simulink model "untitled"  (R2021a)
settings: Solver=VariableStepAuto  StartTime=0.0  StopTime=10.0  RelTol=1e-3
values from neighbouring files (symbols this model uses):
  B = inv(N)    [Para.m]    (also in Parameters.m = inv(N)*[zeros(3);eye(3)])
  dtheta_LMO = sqrt(muy/r_LMO^3)    [Para.m]    (also in Parameters.m)
  hW = [0 h2 0]'    [Para.m]
  I = [10 0 0;0 5 0;0 0 7.5]    [Para.m]    (also in Parameters.m = diag([5 3 6]))
  i0_LMO = pi/6    (= 0.523598775598)    [Para.m]    (also in Parameters.m)
  K = 5    [Para.m]    (also in Parameters.m)
  N = [eye(3) zeros(3);zeros(3) J]    [Dynamics.m]    (also in Para.m; Parameters.m)
  Omega0_LMO = pi/9    (= 0.349065850399)    [Para.m]    (also in Parameters.m)
  P = 10*eye(3)    [Para.m]    (also in Parameters.m)
  R = eye(6)    [Para.m]    (also in Parameters.m = eye(3))
  S = [0 0 0 0.5 0 0;           0 0 0 0 0.5 0;           0 0 0 0 0 0.5;           f41 0 0 0 0 f46;           0 f52 0 0 0 0;           0 0 f63 f64 0 0]    [Para.m]    (also in Parameters.m; crossMatrix.m = [0 -q3 q2;           q3 0 -q1;           -q2 q1 0])
  theta0_LMO = pi/3    (= 1.0471975512)    [Para.m]    (also in Parameters.m)
undefined symbols (not defined in the file or in its folder): F
settings Model: Creator=VTX  LastModifiedBy=VTX

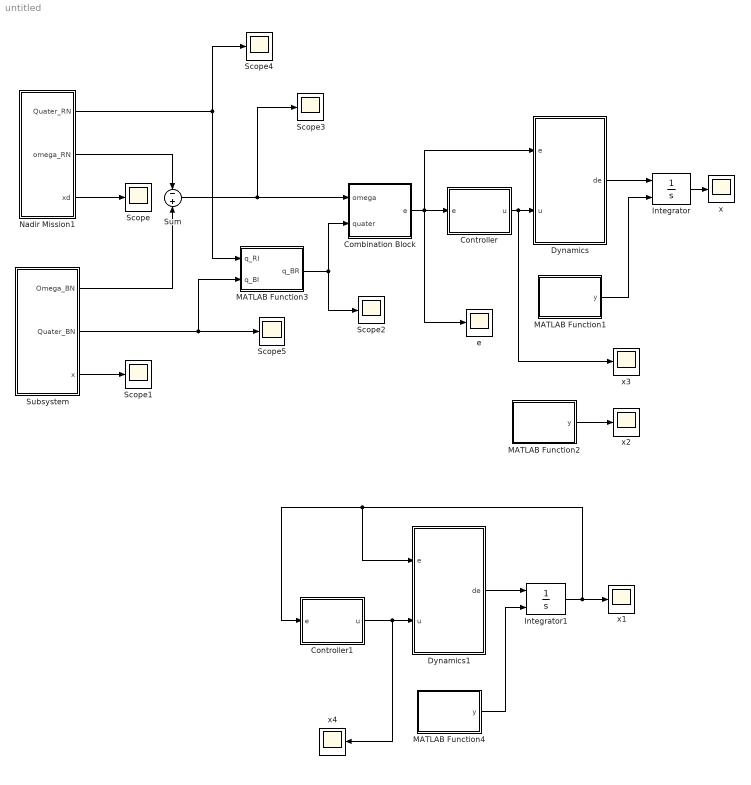
== system untitled ==
  Combination Block : Subsystem
  Controller : MATLAB Function  TreatAsAtomicUnit=on
  Controller1 : MATLAB Function  TreatAsAtomicUnit=on
  Dynamics : MATLAB Function  TreatAsAtomicUnit=on
  Dynamics1 : MATLAB Function  TreatAsAtomicUnit=on
  Integrator : Integrator  InitialConditionSource=external
  Integrator1 : Integrator  InitialConditionSource=external
  MATLAB Function1 : MATLAB Function  TreatAsAtomicUnit=on
  MATLAB Function2 : MATLAB Function  TreatAsAtomicUnit=on
  MATLAB Function3 : MATLAB Function  TreatAsAtomicUnit=on
  MATLAB Function4 : MATLAB Function  TreatAsAtomicUnit=on
  Nadir Mission1 : Subsystem
  Scope{,1..5} (6 alike) : Scope
  Subsystem : Subsystem
  Sum : Sum  Inputs=-|+
  e : Scope
  x{,1..4} (5 alike) : Scope
  wires:
  MATLAB Function2/1(y) -> x2/1
  Integrator1/1 -> Dynamics1/1(e), Controller1/1(e), x1/1
  Dynamics1/1(de) -> Integrator1/1
  MATLAB Function4/1(y) -> Integrator1/2
  Combination Block/1(e) -> e/1, Dynamics/1(e), Controller/1(e)
  Subsystem/1(Omega_BN) -> Sum/2
  Sum/1 -> Combination Block/1(omega), Scope3/1
  Controller1/1(u) -> x4/1, Dynamics1/2(u)
  Dynamics/1(de) -> Integrator/1
  Subsystem/3(x) -> Scope1/1
  MATLAB Function1/1(y) -> Integrator/2
  Nadir Mission1/3(xd) -> Scope/1
  Nadir Mission1/2(omega_RN) -> Sum/1
  Controller/1(u) -> x3/1, Dynamics/2(u)
  Integrator/1 -> x/1
  MATLAB Function3/1(q_BR) -> Combination Block/2(quater), Scope2/1
  Subsystem/2(Quater_BN) -> MATLAB Function3/2(q_BI), Scope5/1
  Nadir Mission1/1(Quater_RN) -> Scope4/1, MATLAB Function3/1(q_RI)

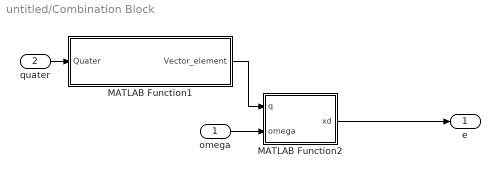
== system untitled/Combination Block ==
  omega : Inport
  quater : Inport  Port=2
  MATLAB Function1 : MATLAB Function  TreatAsAtomicUnit=on
  MATLAB Function2 : MATLAB Function  TreatAsAtomicUnit=on
  e : Outport
  wires:
  MATLAB Function2/1(xd) -> e/1
  MATLAB Function1/1(Vector_element) -> MATLAB Function2/1(q)
  quater/1 -> MATLAB Function1/1(Quater)
  omega/1 -> MATLAB Function2/2(omega)

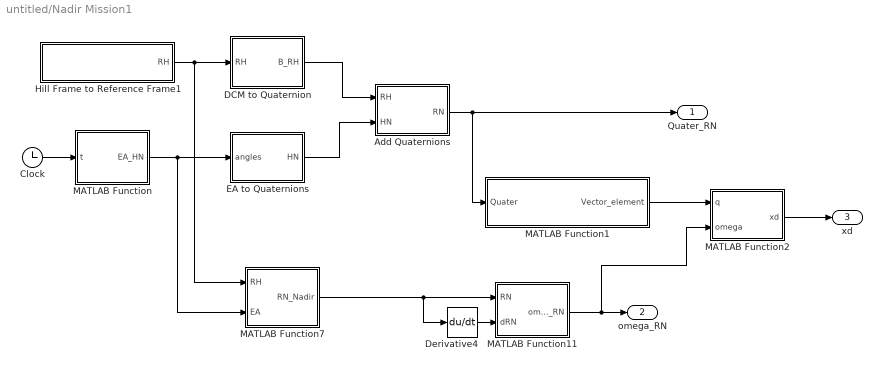
== system untitled/Nadir Mission1 ==
  Add Quaternions : MATLAB Function  TreatAsAtomicUnit=on
  Clock : Clock
  DCM to Quaternion : MATLAB Function  TreatAsAtomicUnit=on
  Derivative4 : Derivative
  EA to Quaternions : MATLAB Function  TreatAsAtomicUnit=on
  Hill Frame to Reference Frame1 : MATLAB Function  TreatAsAtomicUnit=on
  MATLAB Function : MATLAB Function  TreatAsAtomicUnit=on
  MATLAB Function1 : MATLAB Function  TreatAsAtomicUnit=on
  MATLAB Function11 : MATLAB Function  TreatAsAtomicUnit=on
  MATLAB Function2 : MATLAB Function  TreatAsAtomicUnit=on
  MATLAB Function7 : MATLAB Function  TreatAsAtomicUnit=on
  Quater_RN : Outport
  omega_RN : Outport  Port=2
  xd : Outport  Port=3
  wires:
  Hill Frame to Reference Frame1/1(RH) -> MATLAB Function7/1(RH), DCM to Quaternion/1(RH)
  MATLAB Function/1(EA_HN) -> MATLAB Function7/2(EA), EA to Quaternions/1(angles)
  Clock/1 -> MATLAB Function/1(t)
  DCM to Quaternion/1(B_RH) -> Add Quaternions/1(RH)
  EA to Quaternions/1(HN) -> Add Quaternions/2(HN)
  Add Quaternions/1(RN) -> MATLAB Function1/1(Quater), Quater_RN/1
  MATLAB Function7/1(RN_Nadir) -> Derivative4/1, MATLAB Function11/1(RN)
  Derivative4/1 -> MATLAB Function11/2(dRN)
  MATLAB Function11/1(omega_RN) -> MATLAB Function2/2(omega), omega_RN/1
  MATLAB Function1/1(Vector_element) -> MATLAB Function2/1(q)
  MATLAB Function2/1(xd) -> xd/1

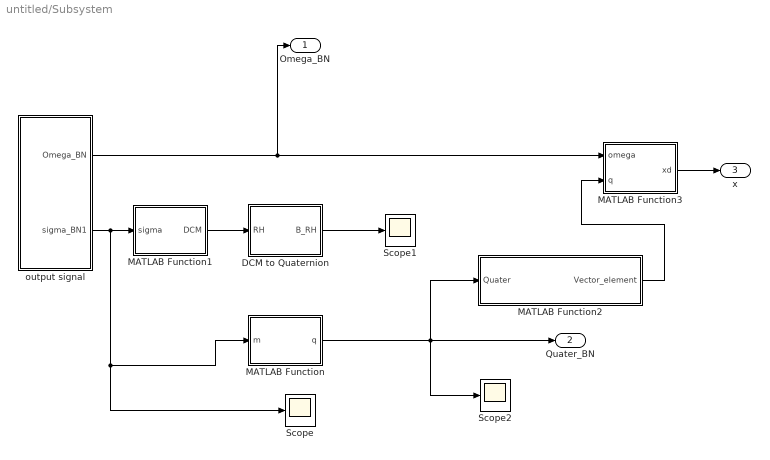
== system untitled/Subsystem ==
  DCM to Quaternion : MATLAB Function  TreatAsAtomicUnit=on
  MATLAB Function : MATLAB Function  TreatAsAtomicUnit=on
  MATLAB Function1 : MATLAB Function  TreatAsAtomicUnit=on
  MATLAB Function2 : MATLAB Function  TreatAsAtomicUnit=on
  MATLAB Function3 : MATLAB Function  TreatAsAtomicUnit=on
  Scope : Scope
  Scope1 : Scope
  Scope2 : Scope
  output signal : Subsystem
  Omega_BN : Outport
  Quater_BN : Outport  Port=2
  x : Outport  Port=3
  wires:
  MATLAB Function1/1(DCM) -> DCM to Quaternion/1(RH)
  MATLAB Function2/1(Vector_element) -> MATLAB Function3/2(q)
  MATLAB Function3/1(xd) -> x/1
  output signal/1(Omega_BN) -> Omega_BN/1, MATLAB Function3/1(omega)
  output signal/2(sigma_BN1) -> MATLAB Function/1(m), Scope/1, MATLAB Function1/1(sigma)
  MATLAB Function/1(q) -> Scope2/1, MATLAB Function2/1(Quater), Quater_BN/1
  DCM to Quaternion/1(B_RH) -> Scope1/1

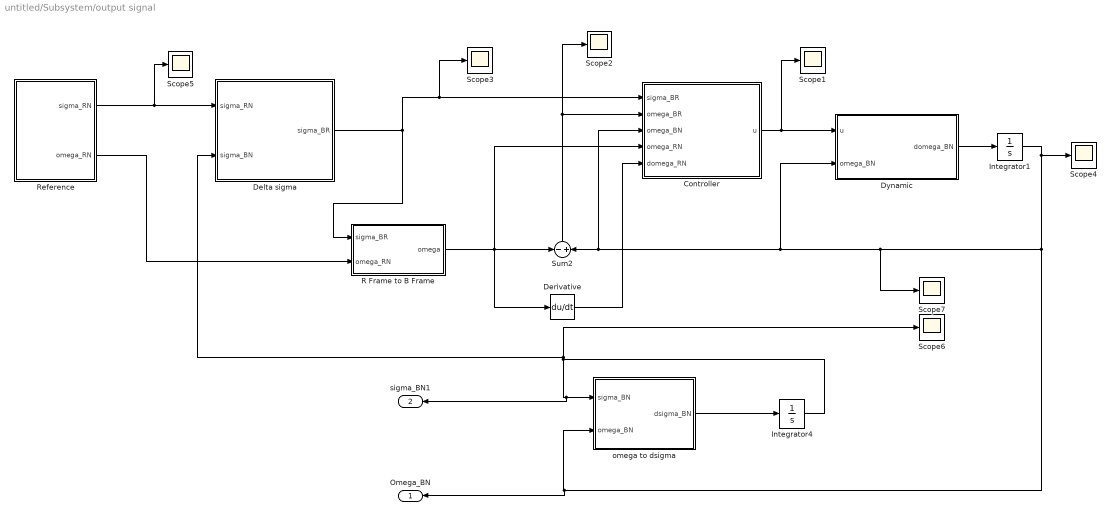
== system untitled/Subsystem/output signal ==
  Controller : MATLAB Function  TreatAsAtomicUnit=on
  Delta sigma : Subsystem
  Derivative : Derivative
  Dynamic : MATLAB Function  TreatAsAtomicUnit=on
  Integrator1 : Integrator  InitialCondition=[1;1.75;-2.2]*pi/180
  Integrator4 : Integrator  InitialCondition=[0.3;-0.4;0.5]
  R Frame to B Frame : MATLAB Function  TreatAsAtomicUnit=on
  Reference : Subsystem
  Scope{1..7} (7 alike) : Scope
  Sum2 : Sum  Inputs=-|+
  omega to dsigma : MATLAB Function  TreatAsAtomicUnit=on
  Omega_BN : Outport
  sigma_BN1 : Outport  Port=2
  wires:
  Derivative/1 -> Controller/5(domega_RN)
  Integrator4/1 -> Scope6/1, Delta sigma/2(sigma_BN), sigma_BN1/1, omega to dsigma/1(sigma_BN)
  Delta sigma/1(sigma_BR) -> Scope3/1, Controller/1(sigma_BR), R Frame to B Frame/1(sigma_BR)
  Dynamic/1(domega_BN) -> Integrator1/1
  Reference/1(sigma_RN) -> Scope5/1, Delta sigma/1(sigma_RN)
  Controller/1(u) -> Scope1/1, Dynamic/1(u)
  Sum2/1 -> Scope2/1, Controller/2(omega_BR)
  Integrator1/1 -> Scope7/1, Dynamic/2(omega_BN), Controller/3(omega_BN), Sum2/2, Omega_BN/1, omega to dsigma/2(omega_BN), Scope4/1
  omega to dsigma/1(dsigma_BN) -> Integrator4/1
  Reference/2(omega_RN) -> R Frame to B Frame/2(omega_RN)
  R Frame to B Frame/1(omega) -> Sum2/1, Derivative/1, Controller/4(omega_RN)

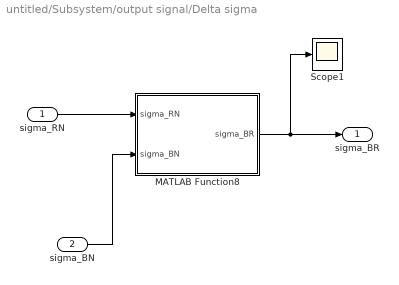
== system untitled/Subsystem/output signal/Delta sigma ==
  sigma_RN : Inport
  sigma_BN : Inport  Port=2
  MATLAB Function8 : MATLAB Function  TreatAsAtomicUnit=on
  Scope1 : Scope
  sigma_BR : Outport
  wires:
  sigma_BN/1 -> MATLAB Function8/2(sigma_BN)
  MATLAB Function8/1(sigma_BR) -> Scope1/1, sigma_BR/1
  sigma_RN/1 -> MATLAB Function8/1(sigma_RN)

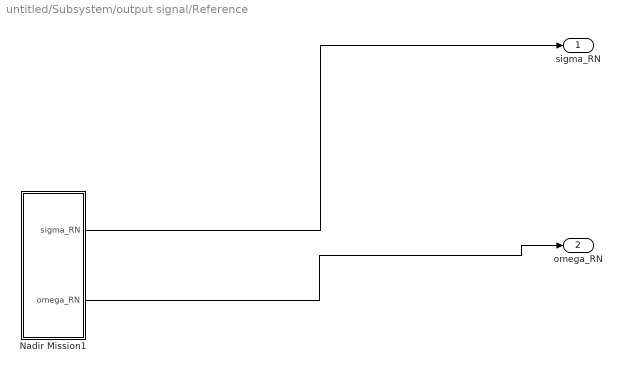
== system untitled/Subsystem/output signal/Reference ==
  Nadir Mission1 : Subsystem
  sigma_RN : Outport
  omega_RN : Outport  Port=2
  wires:
  Nadir Mission1/2(omega_RN) -> omega_RN/1
  Nadir Mission1/1(sigma_RN) -> sigma_RN/1

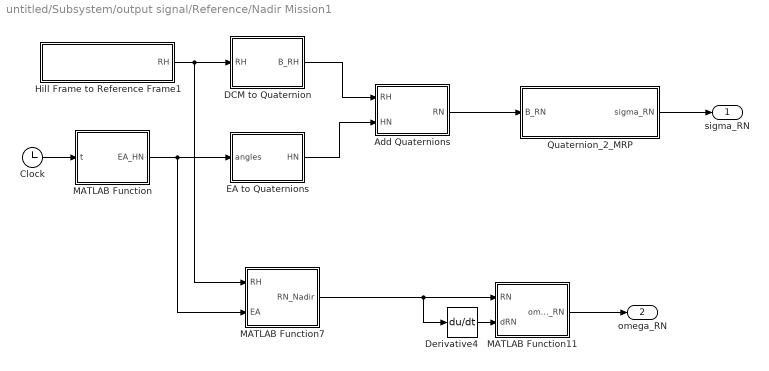
== system untitled/Subsystem/output signal/Reference/Nadir Mission1 ==
  Add Quaternions : MATLAB Function  TreatAsAtomicUnit=on
  Clock : Clock
  DCM to Quaternion : MATLAB Function  TreatAsAtomicUnit=on
  Derivative4 : Derivative
  EA to Quaternions : MATLAB Function  TreatAsAtomicUnit=on
  Hill Frame to Reference Frame1 : MATLAB Function  TreatAsAtomicUnit=on
  MATLAB Function : MATLAB Function  TreatAsAtomicUnit=on
  MATLAB Function11 : MATLAB Function  TreatAsAtomicUnit=on
  MATLAB Function7 : MATLAB Function  TreatAsAtomicUnit=on
  Quaternion_2_MRP : MATLAB Function  TreatAsAtomicUnit=on
  sigma_RN : Outport
  omega_RN : Outport  Port=2
  wires:
  Hill Frame to Reference Frame1/1(RH) -> MATLAB Function7/1(RH), DCM to Quaternion/1(RH)
  MATLAB Function/1(EA_HN) -> MATLAB Function7/2(EA), EA to Quaternions/1(angles)
  Clock/1 -> MATLAB Function/1(t)
  DCM to Quaternion/1(B_RH) -> Add Quaternions/1(RH)
  EA to Quaternions/1(HN) -> Add Quaternions/2(HN)
  Add Quaternions/1(RN) -> Quaternion_2_MRP/1(B_RN)
  Quaternion_2_MRP/1(sigma_RN) -> sigma_RN/1
  MATLAB Function7/1(RN_Nadir) -> Derivative4/1, MATLAB Function11/1(RN)
  Derivative4/1 -> MATLAB Function11/2(dRN)
  MATLAB Function11/1(omega_RN) -> omega_RN/1

== matlab function untitled/Nadir Mission1/Add Quaternions ==
  data: RH input; RN output; HN input
function RN = f(RH,HN)
    %% [BN] = [BR]*[RN]
    q0 = RH(1);
    q1 = RH(2);
    q2 = RH(3);
    q3 = RH(4);
    
    Matrix = [q0 -q1 -q2 -q3; ...
              q1 q0 q3 -q2; ...
              q2 -q3 q0 q1; ...
              q3 q2 -q1 q0];
    RN = Matrix*HN;
end

== matlab function untitled/Nadir Mission1/DCM to Quaternion ==
  data: RH input; B_RH output size=4
function B_RH = fcn(RH)
    trace = RH(1,1) + RH(2,2) + RH(3,3);
    beta0 = (0.25*(1 + trace));
    beta1 = (0.25*(1 + 2*RH(1,1) - trace));
    beta2 = (0.25*(1 + 2*RH(2,2) - trace));
    beta3 = (0.25*(1 + 2*RH(3,3) - trace));
    
    m = max([beta0 beta1 beta2 beta3]);

    B0 = 0; B1 = 0; B2 = 0; B3 = 0;
    
    if beta0 == m
        B0 = sqrt(beta0);
        B1 = (RH(2,3)-RH(3,2))/(4*B0);
        B2 = (RH(3,1)-RH(1,3))/(4*B0);
        B3 = (RH(1,2)-RH(2,1))/(4*B0);
    elseif beta1 == m
        B1 = sqrt(beta1);
        B0 = (RH(2,3)-RH(3,2))/(4*B1);
        B2 = (RH(1,2)+RH(2,1))/(4*B1);
        B3 = (RH(3,1)+RH(1,3))/(4*B1);
    elseif beta2 == m
        B2 = sqrt(beta2);
        B0 = (RH(3,1)-RH(1,3))/(4*B2);
        B1 = (RH(1,2)+RH(2,1))/(4*B2);
        B3 = (RH(2,3)+RH(3,2))/(4*B2);
    elseif beta3 == m
        B3 = sqrt(beta3);
        B0 = (RH(1,2)-RH(2,1))/(4*B3);
        B1 = (RH(3,1)+RH(1,3))/(4*B3);
        B2 = (RH(2,3)+RH(3,2))/(4*B3);
    end
    
    B_RH = [B0 B1 B2 B3]';
end

== matlab function untitled/Nadir Mission1/EA to Quaternions ==
  data: angles input; HN output
function HN = EulerAngles313_2_Quaternions(angles)
    Omega = angles(1);
    i = angles(2);
    omega = angles(3);

    q0 = cos(omega/2)*cos(i/2)*cos(Omega/2) - sin(omega/2)*cos(i/2)*sin(Omega/2);
    q1 = cos(omega/2)*sin(i/2)*cos(Omega/2) + sin(omega/2)*sin(i/2)*sin(Omega/2);
    q2 = -sin(omega/2)*sin(i/2)*cos(Omega/2) + cos(omega/2)*sin(i/2)*sin(Omega/2);
    q3 = sin(omega/2)*cos(i/2)*cos(Omega/2) + cos(omega/2)*cos(i/2)*sin(Omega/2);
    
    HN = [q0 q1 q2 q3]';
end

== matlab function untitled/Subsystem/output signal/Reference/Nadir Mission1/Hill Frame to Reference Frame1 ==
  data: RH output
function RH = fcn()
RH = [-1 0 0;0 1 0;0 0 -1];
end

== matlab function untitled/Subsystem/output signal/Reference/Nadir Mission1/MATLAB Function ==
  data: t input; EA_HN output; Omega0_LMO parameter; i0_LMO parameter; theta0_LMO parameter; dtheta_LMO parameter
function EA_HN = fcn(t,Omega0_LMO, i0_LMO, theta0_LMO, dtheta_LMO)
    EA_HN = [Omega0_LMO i0_LMO (theta0_LMO + dtheta_LMO*t)]';
end

== matlab function untitled/Subsystem/output signal/Reference/Nadir Mission1/MATLAB Function11 ==
  data: RN input; omega_RN output; dRN input
function omega_RN = fcn(RN,dRN)
    omega_RN_tidle = -dRN*RN';
    o1 = omega_RN_tidle(3,2);
    o2 = omega_RN_tidle(1,3);
    o3 = omega_RN_tidle(2,1);
    omega_RN = [o1 o2 o3]';
end

== matlab function untitled/Controller ==
  data: e input; u output; F parameter; B parameter; R parameter
function u = fcn(e, F, B, R)
%% Controller
   u = -inv(R)*B'*F*e;
end

== matlab function untitled/Subsystem/output signal/Reference/Nadir Mission1/MATLAB Function7 ==
  data: RN_Nadir output; RH input; EA input
function RN_Nadir  = fcn(RH,EA)
    Omega = EA(1);
    i = EA(2);
    theta = EA(3);

    %% Rotate about z axis
    Cz1 = [cos(Omega) sin(Omega) 0;-sin(Omega) cos(Omega) 0;0 0 1];

    %% Rotate about x axis
    Cx2 = [1 0 0;0 cos(i) sin(i);0 -sin(i) cos(i)];
    
    %% Rotate about z axis
    Cz3 = [cos(theta) sin(theta) 0;-sin(theta) cos(theta) 0;0 0 1];

    %% DCM from Inertial Frame to Hill Frame
    HN = Cz3*Cx2*Cz1;
    
    %% DCm from Inertial Frame to Reference Frame
    RN_Nadir = RH*HN;
end

== matlab function untitled/Subsystem/output signal/Reference/Nadir Mission1/Quaternion_2_MRP ==
  data: B_RN input; sigma_RN output
function sigma_RN  = fcn(B_RN)
    sigma1 = B_RN(2)/(1 + B_RN(1));
    sigma2 = B_RN(3)/(1 + B_RN(1));
    sigma3 = B_RN(4)/(1 + B_RN(1));
    
    sigma_RN = [sigma1 sigma2 sigma3]';
end

== matlab function untitled/Nadir Mission1/Hill Frame to Reference Frame1 ==
  data: RH output
function RH = fcn()
RH = [-1 0 0;0 1 0;0 0 -1];
end

== matlab function untitled/Nadir Mission1/MATLAB Function ==
  data: t input; EA_HN output; Omega0_LMO parameter; i0_LMO parameter; theta0_LMO parameter; dtheta_LMO parameter
function EA_HN = fcn(t,Omega0_LMO, i0_LMO, theta0_LMO, dtheta_LMO)
    EA_HN = [Omega0_LMO i0_LMO (theta0_LMO + dtheta_LMO*t)]';
end

== matlab function untitled/Nadir Mission1/MATLAB Function11 ==
  data: RN input; omega_RN output; dRN input
function omega_RN = fcn(RN,dRN)
    omega_RN_tidle = -dRN*RN';
    o1 = omega_RN_tidle(3,2);
    o2 = omega_RN_tidle(1,3);
    o3 = omega_RN_tidle(2,1);
    omega_RN = [o1 o2 o3]';
end

== matlab function untitled/Nadir Mission1/MATLAB Function7 ==
  data: RN_Nadir output; RH input; EA input
function RN_Nadir  = fcn(RH,EA)
    Omega = EA(1);
    i = EA(2);
    theta = EA(3);

    %% Rotate about z axis
    Cz1 = [cos(Omega) sin(Omega) 0;-sin(Omega) cos(Omega) 0;0 0 1];

    %% Rotate about x axis
    Cx2 = [1 0 0;0 cos(i) sin(i);0 -sin(i) cos(i)];
    
    %% Rotate about z axis
    Cz3 = [cos(theta) sin(theta) 0;-sin(theta) cos(theta) 0;0 0 1];

    %% DCM from Inertial Frame to Hill Frame
    HN = Cz3*Cx2*Cz1;
    
    %% DCm from Inertial Frame to Reference Frame
    RN_Nadir = RH*HN;
end

== matlab function untitled/Nadir Mission1/MATLAB Function1 ==
  data: Quater input; Vector_element output
function Vector_element = fcn(Quater)
    Vector_element = Quater(2:4);
end

== matlab function untitled/Nadir Mission1/MATLAB Function2 ==
  data: q input; xd output; omega input
function xd = fcn(q,omega)
    xd = [q;omega]; 
end

== matlab function untitled/Subsystem/MATLAB Function1 ==
  data: sigma input; DCM output
function DCM = MRP2DCM(sigma)
    %% This function returns a DCM that is transformed from MRP
    s1 = sigma(1);
    s2 = sigma(2);
    s3 = sigma(3);
    
    sigma_cross = [0 -s3 s2;s3 0 -s1;-s2 s1 0];
    
    DCM = eye(3) + (8*sigma_cross*sigma_cross - 4*(1 - dot(sigma,sigma))*sigma_cross)/(1 + dot(sigma,sigma))^2;

end

== matlab function untitled/Subsystem/DCM to Quaternion ==
  data: RH input; B_RH output size=4
function B_RH = fcn(RH)
    trace = RH(1,1) + RH(2,2) + RH(3,3);
    beta0 = (0.25*(1 + trace));
    beta1 = (0.25*(1 + 2*RH(1,1) - trace));
    beta2 = (0.25*(1 + 2*RH(2,2) - trace));
    beta3 = (0.25*(1 + 2*RH(3,3) - trace));
    
    m = max([beta0 beta1 beta2 beta3]);

    B0 = 0; B1 = 0; B2 = 0; B3 = 0;
    
    if beta0 == m
        B0 = sqrt(beta0);
        B1 = (RH(2,3)-RH(3,2))/(4*B0);
        B2 = (RH(3,1)-RH(1,3))/(4*B0);
        B3 = (RH(1,2)-RH(2,1))/(4*B0);
    elseif beta1 == m
        B1 = sqrt(beta1);
        B0 = (RH(2,3)-RH(3,2))/(4*B1);
        B2 = (RH(1,2)+RH(2,1))/(4*B1);
        B3 = (RH(3,1)+RH(1,3))/(4*B1);
    elseif beta2 == m
        B2 = sqrt(beta2);
        B0 = (RH(3,1)-RH(1,3))/(4*B2);
        B1 = (RH(1,2)+RH(2,1))/(4*B2);
        B3 = (RH(2,3)+RH(3,2))/(4*B2);
    elseif beta3 == m
        B3 = sqrt(beta3);
        B0 = (RH(1,2)-RH(2,1))/(4*B3);
        B1 = (RH(3,1)+RH(1,3))/(4*B3);
        B2 = (RH(2,3)+RH(3,2))/(4*B3);
    end
    
    B_RH = [B0 B1 B2 B3]';
end

== matlab function untitled/Subsystem/MATLAB Function2 ==
  data: Quater input; Vector_element output
function Vector_element = fcn(Quater)
    Vector_element = Quater(2:4);
end

== matlab function untitled/Subsystem/output signal/Delta sigma/MATLAB Function8 ==
  data: sigma_BR output; sigma_RN input; sigma_BN input
function sigma_BR = fcn(sigma_RN, sigma_BN)
    sigma_BR = ((1 - norm(sigma_RN)^2)*sigma_BN - (1 - norm(sigma_BN)^2)*sigma_RN + 2*cross(sigma_BN,sigma_RN))/(1 + norm(sigma_RN)^2*norm(sigma_BN)^2 + 2*dot(sigma_RN,sigma_BN));
end

== matlab function untitled/Subsystem/MATLAB Function3 ==
  data: omega input; q input; xd output
function xd = fcn(omega, q)
    xd = [q;omega]; 
end

== matlab function untitled/Dynamics ==
  data: e input; de output; u input; N parameter; S parameter
function de  = fcn(e,u,N,S)
%% Quaternions
    %q = [q1 q2 q3]';
    %quater = [q0 q']';

%% State Model: dx = Ax + Bu
    %dx = inv(N)*(S*[q' omega_BR']' + [0 0 0 u']');
    %de = inv(N)*(S*e + [0 0 0 u']');
    de = inv(N)*(S*e + u);
end

== matlab function untitled/Combination Block/MATLAB Function1 ==
  data: Quater input; Vector_element output
function Vector_element = fcn(Quater)
    Vector_element = Quater(2:4);
end

== matlab function untitled/Combination Block/MATLAB Function2 ==
  data: q input; xd output; omega input
function xd = fcn(q,omega)
    xd = [q;omega]; 
end

== matlab function untitled/Subsystem/MATLAB Function ==
  data: m input; q output
function q = mrp2quat(m)

  m=m(:);
  magsq=m'*m;
  q=[(1 - magsq); 2*m(1:3)]./(1 + magsq);
   
return

== matlab function untitled/Subsystem/output signal/omega to dsigma ==
  data: sigma_BN input; dsigma_BN output size=3; omega_BN input
function dsigma_BN = fcn(sigma_BN,omega_BN)
   sigma_tilde = [0 -sigma_BN(3) sigma_BN(2);sigma_BN(3) 0 -sigma_BN(1);-sigma_BN(2) sigma_BN(1) 0];
   dsigma_BN = 1/4*((1 - dot(sigma_BN,sigma_BN))*eye(3) + 2*sigma_tilde + 2*sigma_BN*sigma_BN')*omega_BN;
end

== matlab function untitled/Controller1 ==
  data: e input; u output; F parameter; B parameter; R parameter
function u = fcn(e, F, B, R)
%% Controller
   u = -inv(R)*B'*F*e;
end

== matlab function untitled/Dynamics1 ==
  data: e input; de output; u input; N parameter; S parameter
function de  = fcn(e,u,N,S)
%% Quaternions
    %q = [q1 q2 q3]';
    %quater = [q0 q']';

%% State Model: dx = Ax + Bu
    %dx = inv(N)*(S*[q' omega_BR']' + [0 0 0 u']');
    %de = inv(N)*(S*e + [0 0 0 u']');
    de = inv(N)*(S*e + u);
end

== matlab function untitled/MATLAB Function1 ==
  data: y output
function y = fcn()
    y = [0.380636677657970 0.805066318975925 0.0572178012633585 -0.0174532925199433 -0.0305432619099008 0.0383972435438753]';
end

== matlab function untitled/MATLAB Function2 ==
  data: y output
function y = fcn()
    k = [4 0 7];
    k = k/norm(k);
    
    y = [sin(pi/10)*k rand(1,3)]';
end

== matlab function untitled/MATLAB Function4 ==
  data: y output
function y = fcn()
    y = [0.380636677657970 0.805066318975925 0.0572178012633585 -0.0174532925199433 -0.0305432619099008 0.0383972435438753]';
end

== matlab function untitled/Subsystem/output signal/Controller ==
  data: sigma_BR input; u output; omega_BR input; K parameter; P parameter; omega_BN input; omega_RN input; I parameter; domega_RN input
function u = fcn(sigma_BR,omega_BR,K,P,omega_BN,omega_RN, I,domega_RN)

    u = -K*sigma_BR - P*omega_BR;
    % u = -K*sigma_BR - P*omega_BR + I*(domega_RN - cross(omega_BN,omega_RN)) + cross(omega_BN,(I*omega_BN));
end

== matlab function untitled/Subsystem/output signal/Dynamic ==
  data: u input; domega_BN output size=3; omega_BN input; I parameter; hW parameter
function domega_BN = fcn(u,omega_BN, I, hW)
    domega_BN = inv(I)*(-cross(omega_BN,(I*omega_BN)) - cross(omega_BN,hW) + u);
end

== matlab function untitled/MATLAB Function3 ==
  data: q_RI input; q_BR output; q_BI input
function q_BR = fcn(q_RI,q_BI)
    %% [RI]=[RB].[BI]
    B0 = q_BI(1);
    B1 = q_BI(2);
    B2 = q_BI(3);
    B3 = q_BI(4);
    
    Matrix = [B0 -B1 -B2 -B3; ...
              B1 B0 -B3 B2; ...
              B2 B3 B0 -B1; ...
              B3 -B2 B1 B0];
    q_RB = inv(Matrix)*q_RI;
    q_BR = [q_RB(1);-q_RB(2:4)];
end

== matlab function untitled/Subsystem/output signal/R Frame to B Frame ==
  data: omega output; sigma_BR input; omega_RN input
function omega = fcn(sigma_BR, omega_RN)
    %% This function returns a DCM that is transformed from MRP
    s1 = sigma_BR(1);
    s2 = sigma_BR(2);
    s3 = sigma_BR(3);
    
    sigma_cross = [0 -s3 s2;s3 0 -s1;-s2 s1 0];
    
    DCM = eye(3) + (8*sigma_cross*sigma_cross - 4*(1 - dot(sigma_BR,sigma_BR))*sigma_cross)/(1 + dot(sigma_BR,sigma_BR))^2;
    
    omega  = DCM*omega_RN;
end

== matlab function untitled/Subsystem/output signal/Reference/Nadir Mission1/Add Quaternions ==
  data: RH input; RN output; HN input
function RN = f(RH,HN)
    %% [BN] = [BR]*[RN]
    q0 = RH(1);
    q1 = RH(2);
    q2 = RH(3);
    q3 = RH(4);
    
    Matrix = [q0 -q1 -q2 -q3; ...
              q1 q0 q3 -q2; ...
              q2 -q3 q0 q1; ...
              q3 q2 -q1 q0];
    RN = Matrix*HN;
end

== matlab function untitled/Subsystem/output signal/Reference/Nadir Mission1/DCM to Quaternion ==
  data: RH input; B_RH output size=4
function B_RH = fcn(RH)
    trace = RH(1,1) + RH(2,2) + RH(3,3);
    beta0 = (0.25*(1 + trace));
    beta1 = (0.25*(1 + 2*RH(1,1) - trace));
    beta2 = (0.25*(1 + 2*RH(2,2) - trace));
    beta3 = (0.25*(1 + 2*RH(3,3) - trace));
    
    m = max([beta0 beta1 beta2 beta3]);

    B0 = 0; B1 = 0; B2 = 0; B3 = 0;
    
    if beta0 == m
        B0 = sqrt(beta0);
        B1 = (RH(2,3)-RH(3,2))/(4*B0);
        B2 = (RH(3,1)-RH(1,3))/(4*B0);
        B3 = (RH(1,2)-RH(2,1))/(4*B0);
    elseif beta1 == m
        B1 = sqrt(beta1);
        B0 = (RH(2,3)-RH(3,2))/(4*B1);
        B2 = (RH(1,2)+RH(2,1))/(4*B1);
        B3 = (RH(3,1)+RH(1,3))/(4*B1);
    elseif beta2 == m
        B2 = sqrt(beta2);
        B0 = (RH(3,1)-RH(1,3))/(4*B2);
        B1 = (RH(1,2)+RH(2,1))/(4*B2);
        B3 = (RH(2,3)+RH(3,2))/(4*B2);
    elseif beta3 == m
        B3 = sqrt(beta3);
        B0 = (RH(1,2)-RH(2,1))/(4*B3);
        B1 = (RH(3,1)+RH(1,3))/(4*B3);
        B2 = (RH(2,3)+RH(3,2))/(4*B3);
    end
    
    B_RH = [B0 B1 B2 B3]';
end

== matlab function untitled/Subsystem/output signal/Reference/Nadir Mission1/EA to Quaternions ==
  data: angles input; HN output
function HN = EulerAngles313_2_Quaternions(angles)
    Omega = angles(1);
    i = angles(2);
    omega = angles(3);

    q0 = cos(omega/2)*cos(i/2)*cos(Omega/2) - sin(omega/2)*cos(i/2)*sin(Omega/2);
    q1 = cos(omega/2)*sin(i/2)*cos(Omega/2) + sin(omega/2)*sin(i/2)*sin(Omega/2);
    q2 = -sin(omega/2)*sin(i/2)*cos(Omega/2) + cos(omega/2)*sin(i/2)*sin(Omega/2);
    q3 = sin(omega/2)*cos(i/2)*cos(Omega/2) + cos(omega/2)*cos(i/2)*sin(Omega/2);
    
    HN = [q0 q1 q2 q3]';
end
